simulink model "p1_e2"  (R2023b)
settings: Solver=VariableStepAuto  StartTime=0.0  StopTime=100  RelTol=1e-3
settings Model: LastModifiedBy=enrique

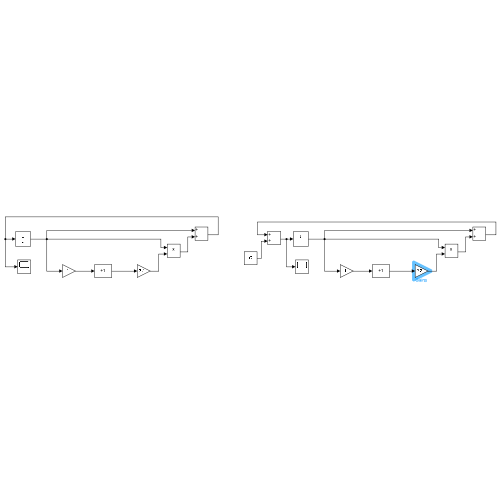
[thumbnail: Simulink's stored preview of the top-level diagram]
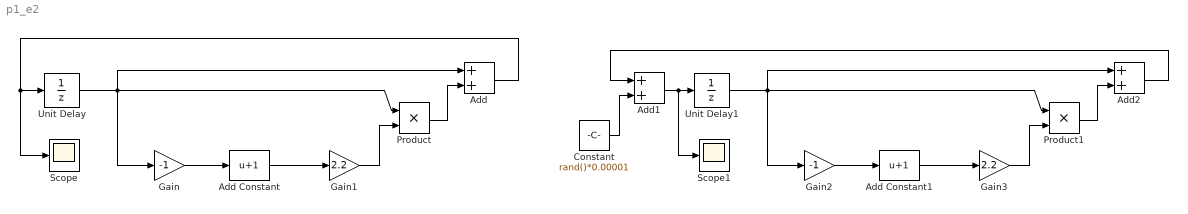
== system p1_e2 ==
  Add : Sum
  Add Constant : Bias  Bias=1  SaturateOnIntegerOverflow=off
  Add Constant1 : Bias  Bias=1  SaturateOnIntegerOverflow=off
  Add1 : Sum
  Add2 : Sum
  Constant : Constant  Value=rand()*0.00001
  Gain : Gain  Gain=-1
  Gain1 : Gain  Gain=2.2
  Gain2 : Gain  Gain=-1
  Gain3 : Gain  Gain=2.2
  Product : Product
  Product1 : Product
  Scope : Scope
  Scope1 : Scope
  Unit Delay : UnitDelay  InitialCondition=rand(5,1)*1.3  SampleTime=-1  HasFrameUpgradeWarning=on
  Unit Delay1 : UnitDelay  InitialCondition=rand(5,1)*1.3  SampleTime=-1  HasFrameUpgradeWarning=on
  wires:
  Add Constant/1 -> Gain1/1
  Gain/1 -> Add Constant/1
  Unit Delay/1 -> Add/1, Gain/1, Product/1
  Gain1/1 -> Product/2
  Product/1 -> Add/2
  Add/1 -> Scope/1, Unit Delay/1
  Gain2/1 -> Add Constant1/1
  Product1/1 -> Add2/2
  Gain3/1 -> Product1/2
  Unit Delay1/1 -> Add2/1, Gain2/1, Product1/1
  Add Constant1/1 -> Gain3/1
  Add2/1 -> Add1/1
  Add1/1 -> Scope1/1, Unit Delay1/1
  Constant/1 -> Add1/2
